simulink model "PMSMdetailTestbench"  (R2022b)
settings: Solver=ode1be  StartTime=0.0  StopTime=400  FixedStep=electricDrive.PmsmControlParams.Ts  RelTol=1e-3  EnableMultiTasking=on
PreLoadFcn:
  | PMSMSystemParamsPopl;
  | load WaterProperties.mat;
  | PMSMthermalParams;
StopFcn:
  | ee_addSimlogTimeStamp(bdroot)
undefined symbols (not defined in the file): electricDrive, p
libraries: fl_lib x71, nesl_utility x25, fl_ps_legacy_lib x23, ee_lib x4, eeTransforms x2, batteryecm_lib x1, autolibshared x1, eePmsmCurrentController x1, eePmsmFwController x1, simulink x1, eePmsmCurrentReferenceGen x1, eeVelocityController x1
(part 1 of 2)
CloseFcn:
  | try,close(h1_ee_pmsm_field_weakening_control),end
  | clear h1_ee_pmsm_field_weakening_control
  | 
  | clear simlogPMSMfocControlLossMaoGen
  | clear logsoutPMSMfocControlLossMaoGen
  | clear air_density alpha beta  Cdc CopperDensity CopperSpHeat CopperThconductivity Cp Cv drag_coefficient dt  gravity h h_conv IronDensity IronSpHeat IronThConductivity Jm k Ld lossMat Lq  max_power max_torque MotorThermal nu p Pmax PmsmControlParams PmsmParams rho  spMat tqMat tout T Tmax  u VehicleParams Vnom
Description:
  | Copyright 2022 - 2023 The MathWorks, Inc.
settings Model: Creator=The MathWorks, Inc.  LastModifiedBy=jjha
settings SolverCC: AlgebraicLoopSolver=TrustRegion  AutoInsertRateTranBlk=on  MaxZcPerStep=1
settings DataIOCC: MaxDataPoints=210000  ReturnWorkspaceOutputs=off  SignalLoggingName=logsoutPMSMfocControlLossMaoGen
settings OptimizationCC: LifeSpan=inf
settings DebuggingCC: UnderspecifiedInitializationDetection=Classic  MergeDetectMultiDrivingBlocksExec=none  UnconnectedInputMsg=warning  UnconnectedOutputMsg=warning  UnconnectedLineMsg=warning  SFUnexpectedBacktrackingDiag=warning  SFNoUnconditionalDefaultTransitionDiag=warning  SFExecutionAtInitializationDiag=none  SFMachineParentedDataDiag=warning  ArithmeticOperatorsInVariantConditions=warning
settings ModelReferenceCC: EnableRefExpFcnMdlSchedulingChecks=on
settings SFSimCC: SimUseLocalCustomCode=off  CustomCodeUndefinedFunction=UseInterfaceOnly
settings RTWCC: RTWUseLocalCustomCode=off  DLArmComputeVersion=19.05
settings CodeAppCC: StateflowObjectComments=on
settings GRTTargetCC: TargetLangStandard=C89/C90 (ANSI)
settings ConfigComp: CovMetricSettings=dw  CovSaveCumulativeToWorkspaceVar=on  CovSaveSingleToWorkspaceVar=on  CovExternalEMLEnable=off
settings SimscapeCC: SimscapeNormalizeSystem=off  SimscapeLogType=all  SimscapeLogSimulationStatistics=on  SimscapeLogName=simlogPMSMdetailTestbench  SimscapeLogDataHistory=700000

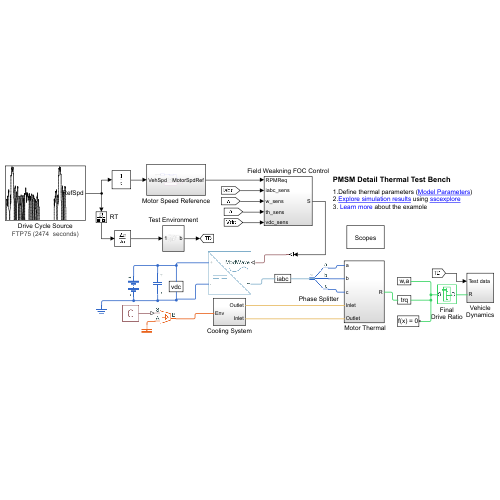
[thumbnail: Simulink's stored preview of the top-level diagram]
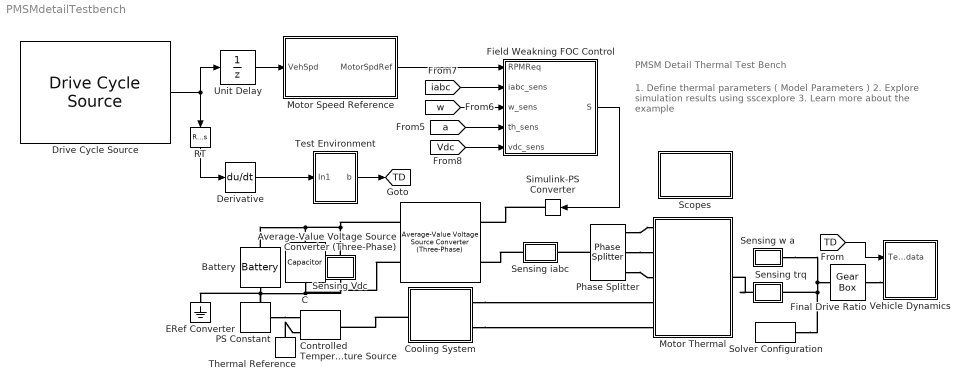
== system PMSMdetailTestbench ==
  note: PMSM Detail Thermal Test Bench
  note: 1. Define thermal parameters ( Model Parameters )
      | 2. Explore simulation results using sscexplore
      | 3. Learn more about the example
  " Motor Thermal" : Subsystem  Tag=PublishSubsystem  VariantControl=Variant1
  Average-Value Voltage Source Converter (Three-Phase) : ee_lib/Semiconductors & Converters/Converters/Average-Value Voltage Source Converter (Three-Phase)  port_option=ee.enum.threePhasePort.composite  frequency_option=ee.enum.converters.frequency.variable  FRated=60 Hz  losses_parameterization=ee.enum.converters.losses.fixed  Pfixed=1 W  ks=0.01  kc1=1.7 V  kc2=0.01 Ohm  Ploss_vect=[100, 800, 1870, 3250, 4900] W  Irms_vect=[10, 100, 200, 300, 400] A  Vdc_nom=300 V  thermal_mass=30000 J/K  temperature_specify=off  temperature_priority=High  temperature=298.15 K  temperature_nominal_specify=off  temperature_nominal_unit=K  temperature_nominal_value=1
      settings: InternalSimscapePortConfiguration="{\"Bottom\":[],\"Left\":[{\"id\":\"ModWave\",\"label\":\"ModWave\",\"type\":\"input\"},{\"id\":\"N\",\"label\":\"~\",\"type\":\"foundation.electrical.three_phase\"}],\"Right\":[{\"id\":\"p\",\"label\":\"+\",\"type\":\"foundation.electrical.electrical\"},{\"id\":\"n\",\"label\":\"-\",\"type\":\"foundation.electrical.electrical\"}],\"Top\":[]}"
  Battery : batteryecm_lib/Battery  Vnom=electricDrive.Vnom V  prm_dir=1  R1_dis=2 Ohm  R1_ch=2 Ohm  R1=0.001 Ohm  prm_AH=simscape.enum.battery.prm_AH.infinite  AH=200 hr*A  V1=290 V  AH1=50 hr*A  prm_R2=1  R2=2000 Ohm  prm_dyn=1  Rp1=0.005 Ohm  tau1=30 s  Rp2=0.005 Ohm  tau2=30 s  Rp3=0.005 Ohm  tau3=30 s  Rp4=0.005 Ohm  tau4=30 s  Rp5=0.005 Ohm  tau5=30 s  prm_fade=1  N_fade=100  AH_fade=45 hr*A  R1_fade=2.02 Ohm  R1_ch_fade=2.02 Ohm  V1_fade=10.35 V  prm_age=1  prm_age_OCV=1  OCV_age=0.9  SOC_age=60  delta_time_age_vec=[0] d  temperature_age_vec=[273] K  OCV_scaling_age=2.2134e6  OCV_offset_age=1.632e6  temp_exp_age=0.515833569 V  t_exp_age=0.75  i_specify=off  i_priority=None  i=0 A  i_nominal_specify=off  i_nominal_unit=A  i_nominal_value=1  v_specify=off  v_priority=None  v=0 V  v_nominal_specify=off  v_nominal_unit=V  v_nominal_value=1  charge_specify=on  charge_priority=High  charge=200 hr*A  charge_nominal_specify=off  charge_nominal_unit=A*hr  charge_nominal_value=1  num_cycles_specify=off  num_cycles_priority=High  num_cycles=0  num_cycles_nominal_specify=off  num_cycles_nominal_unit=1  num_cycles_nominal_value=1  Tmeas=298.15 K  Tmeas_age=298.15 K  Vnom_T2=12 V  R1_T2=2.2 Ohm  R1_T2_dis=2.2 Ohm  R1_T2_ch=2.2 Ohm  V1_T2=11.4 V  R2_T2=2200 Ohm  Rp1_T2=0.005 Ohm  tau1_T2=30 s  Rp2_T2=0.005 Ohm  tau2_T2=30 s  Rp3_T2=0.005 Ohm  tau3_T2=30 s  Rp4_T2=0.005 Ohm  tau4_T2=30 s  Rp5_T2=0.005 Ohm  tau5_T2=30 s  Tmeas2=273.15 K  thermal_mass=30000 J/K  temperature_specify=off  temperature_priority=High  temperature=298.15 K  temperature_nominal_specify=off  temperature_nominal_unit=K  temperature_nominal_value=1
  C : fl_lib/Electrical/Electrical Elements/Capacitor  c=electricDrive.Cdc F  r=1e-6 Ohm  g=0 1/Ohm  i_specify=off  i_priority=None  i=0 A  i_nominal_specify=off  i_nominal_unit=A  i_nominal_value=1  v_specify=off  v_priority=None  v=0 V  v_nominal_specify=off  v_nominal_unit=V  v_nominal_value=1  vc_specify=on  vc_priority=None  vc=electricDrive.Vnom V  vc_nominal_specify=off  vc_nominal_unit=V  vc_nominal_value=1
  Controlled Temperature Source : fl_lib/Thermal/Thermal Sources/Controlled Temperature Source
  Cooling System : Subsystem  Tag=PublishSubsystem
  Derivative : Derivative
  Drive Cycle Source : autolibshared/Drive Cycle Source  cycleVar=FTP75  fileVar=cycleFTP75.mat  tfinal="2474  seconds"  cycleRepeat=off  outAccPort=off  outGearPort=off  gearList=No gear data  t_wot1=5  xdot_woto=0  xdot_wot1=30  t_wot2=20  xdot_wot2=0  t_wotend=30  srcUnit=m/s  outUnit=km/hr  srcAccUnit=m/s/s  outAccUnit=m/s^2  dt=1e-3  aMode=1  faultOption=off  velBnd=2  velBndUnit=mph  inUnit=m/s  timeBnd=1  failOption=off  stopSim=off  maxFaultCnt=10  maxFaultTime=2  maxTotFaultTime=15  traceOption=off  dtTrace=1  traceWindow=10  lastDCname=FTP75  lastOutUnit=mph  lastDT=1e-3  lastTB=1  lastSB=2  forceCalcBound=off
  ERef Converter : fl_lib/Electrical/Electrical Elements/Electrical Reference
  Field Weakning FOC Control : Subsystem
  Final Drive Ratio : fl_lib/Mechanical/Mechanisms/Gear Box  ratio=electricDrive.VehicleParams.Gear_ratio  t_in_specify=off  t_in_priority=High  t_in=0 N*m  t_in_nominal_specify=off  t_in_nominal_unit=N*m  t_in_nominal_value=1  t_out_specify=off  t_out_priority=High  t_out=0 N*m  t_out_nominal_specify=off  t_out_nominal_unit=N*m  t_out_nominal_value=1
  Motor Speed Reference : Subsystem
  PS Constant : fl_lib/Physical Signals/Sources/PS Constant  constant=298.15 K
  Phase Splitter : ee_lib/Connectors & References/Phase Splitter
  RT : RateTransition  OutPortSampleTime=5e-05
  Scopes : Subsystem
      mask Display: disp(get_param(gcb,'Name'))
  Sensing Vdc : Subsystem
      mask Display: disp('vdc')
  Sensing w a : Subsystem
      mask Display: disp('w,a')
  Sensing iabc : Subsystem
      mask Display: disp('iabc')
  Sensing trq : Subsystem
      mask Display: disp('trq')
  Simulink-PS Converter : nesl_utility/Simulink-PS Converter  PhysicalDomain=network_engine_domain  SubClassName=ps_input  LeftPortType=input  RightPortType=output  PseudoPeriodic=off  Frequencies=[]  NoiseDistribution=none  NoiseParameters=[]  Unit=1  AffineConversion=off  FilteringAndDerivatives=provide  SimscapeFilterOrder=1  InputFilterTimeConstant=0.001  UdotUserProvided=0
  Solver Configuration : nesl_utility/Solver Configuration  PhysicalDomain=network_engine_domain  SubClassName=solver  LeftPortType=input  RightPortType=generic  Tones=[]  Harmonics=[]  SimulateNoise=off  Profile=off  UseLocalSampling=off  EnableSwitchedLinearOptims=on  FrequencyDomain=off  UseCCode=off  RelTol=0.001  AbsTol=1e-06  MinStep=1e-09  ToWorkspace=off  RevertToSquareIcSolve=off  NumHomotopyIterations=100  PhasorMode=off  PhasorModeNumHarmonics=1  ConsistencySolver=NEWTON_FTOL  IndexReductionMethod=DerivativeReplacement  DoDC=off  ResidualTolerance=1e-9  ConsistencyTolSource=GLOBAL  ConsistencyAbsTol=0.001  ConsistencyRelTol=0.001  ConsistencyTolFactor=0.001  UseLocalSolver=on  LocalSolverChoice=NE_BACKWARD_EULER_ADVANCER  ResolveIndetEquations=on  FunctionEvalNumThread=1  LocalSolverSampleTime=electricDrive.PmsmControlParams.Ts  DoFixedCost=on  MaxNonlinIter=4  MaxModeIter=2  ComputeImpulses=off  ImpulseIterations=2  LinearAlgebra=auto  LinearAlgebraNumThread=0  EquationFormulation=NE_TIME_EF  DelaysMemoryBudget=1024  AutomaticFiltering=on  FilteringTimeConstant=0.001  PartitionStorageMethod=AS_NEEDED  PartitionMemoryBudget=1024  PartitionMethod=FAST
  Test Environment : Subsystem
  Thermal Reference : fl_lib/Thermal/Thermal Elements/Thermal Reference
  Unit Delay : UnitDelay  SampleTime=-1  HasFrameUpgradeWarning=on
  Vehicle Dynamics : Subsystem
  tag scope: TD=global
  wires:
  Field Weakning FOC Control/1(S) -> Simulink-PS Converter/1
  [Vdc] -> Field Weakning FOC Control/5(vdc_sens)
  [iabc] -> Field Weakning FOC Control/2(iabc_sens)
  [w] -> Field Weakning FOC Control/3(w_sens)
  [a] -> Field Weakning FOC Control/4(th_sens)
  Motor Speed Reference/1(MotorSpdRef) -> Field Weakning FOC Control/1(RPMReq)
  [TD] -> Vehicle Dynamics/1(Test data)
  Drive Cycle Source/1 -> Unit Delay/1, RT/1
  RT/1 -> Derivative/1
  Unit Delay/1 -> Motor Speed Reference/1(VehSpd)
  Derivative/1 -> Test Environment/1(In1)
  Test Environment/1(b) -> [TD]
  connections:
  Sensing Vdc/LConn1 -- Average-Value Voltage Source Converter (Three-Phase)/RConn1 -- Battery/LConn1 -- C/LConn1
  Sensing iabc/LConn1 -- Average-Value Voltage Source Converter (Three-Phase)/LConn2
  Phase Splitter/LConn1 -- Sensing iabc/RConn1
  Sensing trq/LConn1 -- " Motor Thermal"/RConn1
  Battery/RConn1 -- Average-Value Voltage Source Converter (Three-Phase)/RConn2 -- Sensing Vdc/RConn1 -- C/RConn1 -- ERef Converter/LConn1
  Sensing w a/LConn1 -- Solver Configuration/RConn1 -- Sensing trq/RConn1 -- Final Drive Ratio/LConn1
  Phase Splitter/RConn1 -- " Motor Thermal"/LConn1
  Phase Splitter/RConn2 -- " Motor Thermal"/LConn2
  Phase Splitter/RConn3 -- " Motor Thermal"/LConn3
  Final Drive Ratio/RConn1 -- Vehicle Dynamics/LConn1
  Simulink-PS Converter/RConn1 -- Average-Value Voltage Source Converter (Three-Phase)/LConn1
  Cooling System/RConn1 -- " Motor Thermal"/LConn4
  Cooling System/RConn2 -- " Motor Thermal"/LConn5
  Cooling System/LConn1 -- Controlled Temperature Source/LConn1
  PS Constant/RConn1 -- Controlled Temperature Source/RConn1
  Thermal Reference/LConn1 -- Controlled Temperature Source/RConn2

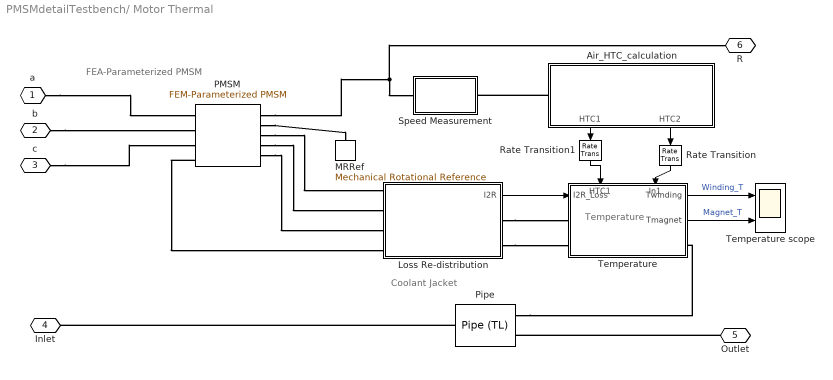
== system PMSMdetailTestbench/ Motor Thermal ==
  note: Temperature
  note: FEA-Parameterized
      | PMSM
  note: Coolant Jacket
  Air_HTC_calculation : Subsystem
      settings: PortSchema="{\"entries\":[{\"content\":{\"sides\":[{\"content\":{\"connectorIds\":[\"LConn1\"]},\"type\":\"ConnectorPlacement.EquallySpacedRectSide\",\"uuid\":\"c3fc49c2-0151-484f-b0d8-f4e4a060bcaf\"},{\"content\":{\"side\":\"RIGHT\"},\"type\":\"ConnectorPlacement.EquallySpacedRectSide\",\"uuid\":\"c73251fe-fcad-4c5f-9d27-fb7ac98c9b31\"},{\"content\":{\"side\":\"TOP\"},\"type\":\"ConnectorPlacement.EquallySpacedRectSide\",\"uuid\":\"06ea8515-c1b4-4445-9ea2-9a6fe3b8d822\"},{\"content\":{\"connectorIds\":[\"Out1\",\"Out2\"],\"side\":\"BOTTOM\"},\"type\":\"ConnectorPlacement.EquallySpacedRectSide\",\"uuid\":\"0d77474d-64a7-49ab-b2b5-eb3962b26dfa\"}]},\"type\":\"ConnectorPlacement.EquallySpacedConnector\",\"uuid\":\"651eda7a-2416-4496-9b8b-1b2d725cf6dd\"}],\"packageUris\":[\"http://schema.mathworks.com/mf0/Connector/R2020b\"],\"version\":\"1.0\"}"
  Loss Re-distribution : Subsystem
  MRRef : fl_lib/Mechanical/Rotational Elements/Mechanical Rotational Reference
  PMSM : ee_lib/Electromechanical/Permanent Magnet/FEM-Parameterized PMSM  parameterization=1  winding_type=ee.enum.statorconnection.wye  iVec=[-2, 0, 2] A  xVec=[0, 20, 40, 60] deg  dfluxdiMatrix=0.0002 * ones(3, 4) Wb/A  dfluxdxMatrix=[0, -.16, .16, 0; 0, -.16, .16, 0; 0, -.16, .16, 0] Wb/rad  calculate_torque_matrix=1  TorqueMatrix=zeros(3, 3, 3, 4) N*m  idVec1=[-200, 0, 200] A  iqVec1=[-200, 0, 200] A  LdMatrix=0.0002 * ones(3, 3) H  LqMatrix=0.0002 * ones(3, 3) H  PmMatrix=0.1 * ones(3, 3) Wb  N=6  interp_method=simscape.enum.interpolation.linear  Rs=electricDrive.PmsmParams.StatorResistance Ohm  Ms=0.00002 H  L0=0.00016 H  loss_param=ee.enum.fem_motor.ironLossesExtended.tabulated  losses_oc=[0, 0, 0] W  losses_sc=[0, 0, 0] W  f_losses=100 % dummy value, not required Hz  Isc_losses=95 A  Inertia=electricDrive.PmsmParams.RotorInertia kg*m^2  lam=0 N*m/(rad/s)  i_d_specify=off  i_d_priority=High  i_d=0 A  i_d_nominal_specify=off  i_d_nominal_unit=A  i_d_nominal_value=1  i_q_specify=off  i_q_priority=High  i_q=0 A  i_q_nominal_specify=off  i_q_nominal_unit=A  i_q_nominal_value=1  torque_specify=off  torque_priority=None  torque=0 N*m  torque_nominal_specify=off  torque_nominal_unit=N*m  torque_nominal_value=1  angular_velocity_specify=off  angular_velocity_priority=High  angular_velocity=PmsmParams.InitialRotorSpeed_rpm rpm  angular_velocity_nominal_specify=off  angular_velocity_nominal_unit=rpm  angular_velocity_nominal_value=1  angular_position_specify=on  angular_position_priority=High  angular_position=electricDrive.PmsmParams.InitialRotorAngle_rad rad  angular_position_nominal_specify=off  angular_position_nominal_unit=deg  angular_position_nominal_value=1  Tmeas=283.15 K  alpha=0.00386 1/K  alpha_flux=-0.001 1/K  stator_thermal_mass=electricDrive.MotorThermal.PhaseWindingThMass J/K  stator_initial_temperatures=[298.15, 298.15, 298.15] K  rotor_thermal_mass=electricDrive.MotorThermal.RotorThMass J/K  rotor_initial_temperature=298.15 K  Rm_percent_rotor=90  Rd_percent_rotor=30  idVec=[-200, 0, 200] A  iqVec=[-200, 0, 200] A  dfluxAdiaMatrix3D=zeros(3, 3, 4) Wb/A  dfluxAdibMatrix3D=zeros(3, 3, 4) Wb/A  dfluxAdicMatrix3D=zeros(3, 3, 4) Wb/A  dfluxAdxMatrix3D=zeros(3, 3, 4) Wb/rad  TorqueMatrix3D=zeros(3, 3, 4) N*m  iaVec=[-200, 0, 200] A  ibVec=[-200, 0, 200] A  icVec=[-200, 0, 200] A  dfluxAdiaMatrix=zeros(3, 3, 3, 4) Wb/A  dfluxAdibMatrix=zeros(3, 3, 3, 4) Wb/A  dfluxAdicMatrix=zeros(3, 3, 3, 4) Wb/A  dfluxAdxMatrix=zeros(3, 3, 3, 4) Wb/rad  param_dq0=ee.enum.fem_motor.fluxTabulationOption.DQpolar  winding_type_dq0=ee.enum.statorconnection.wye  expose_neutral_port=ee.enum.fem_motor.exposeNeutralPort.no  nPolePairs=electricDrive.PmsmParams.NumPolePairs  parks_type=ee.enum.fem_motor.parksType.QleadsD_AphaseToQaxis  idVec2=[-200, 0, 200] A  iqVec2=[-200, 0, 200] A  magVec2=electricDrive.PmsmParams.CurrMagVec*1.3 A  betaVec2=electricDrive.PmsmParams.CurrAdvAngleVec deg  xVec2=electricDrive.PmsmParams.RotorAngleVec deg  fluxD_dq0=zeros(3, 3, 7) Wb  fluxQ_dq0=zeros(3, 3, 7) Wb  fluxA_dq0=zeros(3, 3, 7) Wb  Torque_dq0=zeros(3, 3, 7) N*m  fluxD_IBX=electricDrive.PmsmParams.FluxDMat Wb  fluxQ_IBX=electricDrive.PmsmParams.FluxQMat Wb  fluxA_IBX=fluxAmat Wb  Torque_IBX=electricDrive.PmsmParams.TorqueMat N*m  rotorLossCoeff_k_h_DQ=zeros(3, 3) W/Hz  rotorLossCoeff_k_J_DQ=zeros(3, 3) W/Hz^2  rotorLossCoeff_k_ex_DQ=zeros(3, 3) W/Hz^(3/2)  rotorLossCoeff_k_h_IB=electricDrive.PmsmParams.RotorKhMat W/Hz  rotorLossCoeff_k_J_IB=electricDrive.PmsmParams.RotorKjMat W/Hz^2  rotorLossCoeff_k_ex_IB=electricDrive.PmsmParams.RotorKexMat W/Hz^(3/2)  statorLossCoeff_k_h_DQ=zeros(3, 3) W/Hz  statorLossCoeff_k_J_DQ=zeros(3, 3) W/Hz^2  statorLossCoeff_k_ex_DQ=zeros(3, 3) W/Hz^(3/2)  statorLossCoeff_k_h_IB=electricDrive.PmsmParams.StatorKhMat W/Hz  statorLossCoeff_k_J_IB=electricDrive.PmsmParams.StatorKjMat W/Hz^2  statorLossCoeff_k_ex_IB=electricDrive.PmsmParams.StatorKexMat W/Hz^(3/2)  wVec=[1000, 2000] rpm  rotorLossTable_DQ=zeros(3, 3, 2) W  rotorLossTable_IB=zeros(3, 5, 2) W  statorLossTable_DQ=zeros(3, 3, 2) W  statorLossTable_IB=zeros(3, 5, 2) W  electrical_torque_before_iron_losses_specify=off  electrical_torque_before_iron_losses_priority=None  electrical_torque_before_iron_losses=0 N*m  electrical_torque_before_iron_losses_nominal_specify=off  electrical_torque_before_iron_losses_nominal_unit=N*m  electrical_torque_before_iron_losses_nominal_value=1  Qrotor_specify=off  Qrotor_priority=None  Qrotor=0 J/s  Qrotor_nominal_specify=off  Qrotor_nominal_unit=J/s  Qrotor_nominal_value=1  Qstator_specify=off  Qstator_priority=None  Qstator=0 J/s  Qstator_nominal_specify=off  Qstator_nominal_unit=J/s  Qstator_nominal_value=1
      settings: InternalSimscapePortConfiguration="{\"Bottom\":[],\"Left\":[{\"id\":\"a\",\"label\":\"a\",\"type\":\"foundation.electrical.electrical\"},{\"id\":\"b\",\"label\":\"b\",\"type\":\"foundation.electrical.electrical\"},{\"id\":\"c\",\"label\":\"c\",\"type\":\"foundation.electrical.electrical\"},{\"id\":\"HR\",\"label\":\"HR\",\"type\":\"foundation.thermal.thermal\"}],\"Right\":[{\"id\":\"R\",\"label\":\"R\",\"type\":\"foundation.mechanical.rotational.rotational\"},{\"id\":\"C\",\"label\":\"C\",\"type\":\"foundation.mechanical.rotational.rotational\"},{\"id\":\"HA\",\"label\":\"HA\",\"type\":\"foundation.thermal.thermal\"},{\"id\":\"HB\",\"label\":\"HB\",\"type\":\"foundation.thermal.thermal\"},{\"id\":\"HC\",\"label\":\"HC\",\"type\":\"foundation.thermal.thermal\"}],\"Top\":[]}"
  Pipe : fl_lib/Thermal Liquid/Elements/Pipe (TL)  length=electricDrive.MotorThermal.ChannelLength mm  area=electricDrive.MotorThermal.ChannelSection mm^2  Dh=electricDrive.MotorThermal.ChannelHydraulicdia mm  length_add=500 mm  roughness=1.5e-5 m  Re_lam=2e+3  Re_tur=4e+3  shape_factor=64  Nu_lam=3.66  dynamic_compressibility=1  inertia=0  p0=1 atm  T0=298.15 K  mdot0=0.1 kg/s
  Rate Transition : RateTransition
  Rate Transition1 : RateTransition
  Speed Measurement : Subsystem
  Temperature : Subsystem
      settings: PortSchema="{\"entries\":[{\"content\":{\"sides\":[{\"content\":{\"connectorIds\":[\"In1\",\"LConn1\",\"LConn2\"]},\"type\":\"ConnectorPlacement.EquallySpacedRectSide\",\"uuid\":\"fee72484-960d-4cd4-9296-e38678962aa1\"},{\"content\":{\"connectorIds\":[\"Out1\",\"Out2\",\"RConn1\"],\"side\":\"RIGHT\"},\"type\":\"ConnectorPlacement.EquallySpacedRectSide\",\"uuid\":\"5fc115b4-63fd-47d3-871d-1c82ac52ac43\"},{\"content\":{\"connectorIds\":[\"In2\",\"In3\"],\"side\":\"TOP\"},\"type\":\"ConnectorPlacement.EquallySpacedRectSide\",\"uuid\":\"406f719a-f995-4122-9f35-24e8332a2e84\"},{\"content\":{\"side\":\"BOTTOM\"},\"type\":\"ConnectorPlacement.EquallySpacedRectSide\",\"uuid\":\"14dc85e6-8157-4b38-8651-862ce77721cd\"}]},\"type\":\"ConnectorPlacement.EquallySpacedConnector\",\"uuid\":\"1dcc2b5d-90fd-40de-873d-99118eb86bdd\"}],\"packageUris\":[\"http://schema.mathworks.com/mf0/Connector/R2020b\"],\"version\":\"1.0\"}"
  Temperature scope : Scope  NumInputPorts=2
  a : PMIOPort  Side=Left
  b : PMIOPort  Port=2  Side=Left
  c : PMIOPort  Port=3  Side=Left
  Inlet : PMIOPort  Port=4  Side=Left
  Outlet : PMIOPort  Port=5  Side=Left
  R : PMIOPort  Port=6  Side=Right
  wires:
  Temperature/1(Twinding) -> Temperature scope/1  "Winding_T"
  Temperature/2(Tmagnet) -> Temperature scope/2  "Magnet_T"
  Loss Re-distribution/1(I2R) -> Temperature/1(I2R_Loss)
  Rate Transition/1 -> Temperature/3(In1)
  Air_HTC_calculation/2(HTC2) -> Rate Transition/1
  Air_HTC_calculation/1(HTC1) -> Rate Transition1/1
  Rate Transition1/1 -> Temperature/2(HTC1)
  connections:
  b/RConn1 -- PMSM/LConn2
  Pipe/RConn1 -- Inlet/RConn1
  PMSM/RConn2 -- MRRef/LConn1
  PMSM/RConn1 -- R/RConn1 -- Speed Measurement/LConn1
  Outlet/RConn1 -- Pipe/LConn1
  a/RConn1 -- PMSM/LConn1
  Air_HTC_calculation/LConn1 -- Speed Measurement/RConn1
  Pipe/LConn2 -- Temperature/RConn1
  Loss Re-distribution/RConn1 -- Temperature/LConn1
  Loss Re-distribution/RConn2 -- Temperature/LConn2
  c/RConn1 -- PMSM/LConn3
  PMSM/LConn4 -- Loss Re-distribution/LConn4
  PMSM/RConn3 -- Loss Re-distribution/LConn1
  PMSM/RConn4 -- Loss Re-distribution/LConn2
  PMSM/RConn5 -- Loss Re-distribution/LConn3

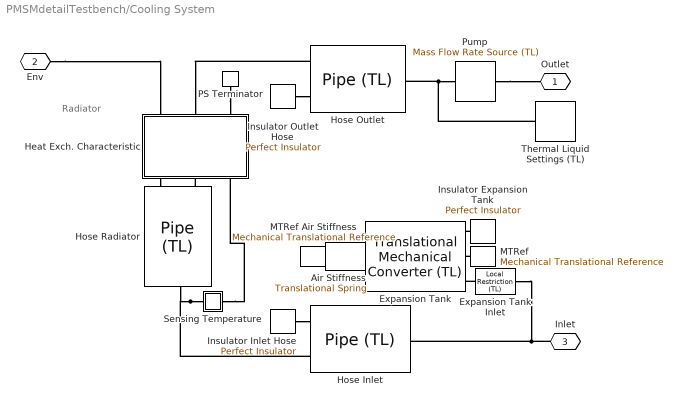
== system PMSMdetailTestbench/Cooling System ==
  note: Radiator
  Air Stiffness : fl_lib/Mechanical/Translational Elements/Translational Spring  spr_rate=1e3 N/m  v_specify=off  v_priority=High  v=0 m/s  v_nominal_specify=off  v_nominal_unit=m/s  v_nominal_value=1  f_specify=on  f_priority=Low  f=0 N  f_nominal_specify=off  f_nominal_unit=N  f_nominal_value=1  x_specify=off  x_priority=High  x=0 m  x_nominal_specify=off  x_nominal_unit=m  x_nominal_value=1
  Expansion Tank : fl_lib/Thermal Liquid/Elements/Translational Mechanical Converter (TL)  mech_orientation=1  displacement_spec=foundation.enum.DisplacementSpec.Calculate  x0=200 mm  interface_area=pi*50^2 mm^2  dead_volume=0.01 m^3  environment_spec=1  environment_pressure=0.101325 MPa  dynamic_compressibility=0  p0=1 atm  T0=298.15 K
      settings: InternalSimscapePortConfiguration="{\"Bottom\":[],\"Left\":[{\"id\":\"A\",\"label\":\"A\",\"type\":\"foundation.thermal_liquid.thermal_liquid\"},{\"id\":\"C\",\"label\":\"C\",\"type\":\"foundation.mechanical.translational.translational\"},{\"id\":\"H\",\"label\":\"H\",\"type\":\"foundation.thermal.thermal\"}],\"Right\":[{\"id\":\"R\",\"label\":\"R\",\"type\":\"foundation.mechanical.translational.translational\"}],\"Top\":[]}"
  Expansion Tank Inlet : fl_lib/Thermal Liquid/Elements/Local Restriction (TL)  restriction_type=foundation.enum.restriction_type.fixed  restriction_area=pi*10^2 mm^2  min_area=1e-10 m^2  max_area=0.005 m^2  area=pi*11^2 mm^2  Cd=0.7  pressure_recovery=0  Re_c=12
  Heat Exch. Characteristic : Subsystem
  Hose Radiator : fl_lib/Thermal Liquid/Elements/Pipe (TL)  length=1000 mm  area=pi*100^2 mm^2  Dh=50 mm  length_add=500 mm  roughness=1.5e-5 m  Re_lam=2e+3  Re_tur=4e+3  shape_factor=64  Nu_lam=3.66  dynamic_compressibility=1  inertia=0  p0=1 atm  T0=298.15 K  mdot0=0.1 kg/s
  Hose Inlet : fl_lib/Thermal Liquid/Elements/Pipe (TL)  length=50 mm  area=pi*100^2 mm^2  Dh=200 mm  length_add=500 mm  roughness=1.5e-5 m  Re_lam=2e+3  Re_tur=4e+3  shape_factor=64  Nu_lam=3.66  dynamic_compressibility=1  inertia=0  p0=1 atm  T0=298.15 K  mdot0=0.1 kg/s
  Hose Outlet : fl_lib/Thermal Liquid/Elements/Pipe (TL)  length=50 mm  area=pi*100^2 mm^2  Dh=200 mm  length_add=500 mm  roughness=1.5e-5 m  Re_lam=2e+3  Re_tur=4e+3  shape_factor=64  Nu_lam=3.66  dynamic_compressibility=1  inertia=0  p0=1 atm  T0=298.15 K  mdot0=0.1 kg/s
  Insulator Expansion Tank : fl_lib/Thermal/Thermal Elements/Perfect Insulator  T_specify=off  T_priority=High  T=0 K  T_nominal_specify=off  T_nominal_unit=K  T_nominal_value=1
  Insulator Inlet Hose : fl_lib/Thermal/Thermal Elements/Perfect Insulator  T_specify=off  T_priority=High  T=0 K  T_nominal_specify=off  T_nominal_unit=K  T_nominal_value=1
  Insulator Outlet Hose : fl_lib/Thermal/Thermal Elements/Perfect Insulator  T_specify=off  T_priority=High  T=0 K  T_nominal_specify=off  T_nominal_unit=K  T_nominal_value=1
  MTRef : fl_lib/Mechanical/Translational Elements/Mechanical Translational Reference
  MTRef Air Stiffness : fl_lib/Mechanical/Translational Elements/Mechanical Translational Reference
  PS Terminator : fl_lib/Physical Signals/Sinks/PS Terminator
  Pump : fl_lib/Thermal Liquid/Sources/Mass Flow Rate Source (TL)  commanded_mass_flow=0.13 kg/s  area=pi*100^2 mm^2
      settings: InternalSimscapePortConfiguration="{\"Bottom\":[],\"Left\":[{\"id\":\"A\",\"label\":\"A\",\"type\":\"foundation.thermal_liquid.thermal_liquid\"}],\"Right\":[{\"id\":\"B\",\"label\":\"B\",\"type\":\"foundation.thermal_liquid.thermal_liquid\"}],\"Top\":[]}"
  Sensing Temperature : Subsystem
      mask Display: disp('T')
  Thermal Liquid Settings (TL) : fl_lib/Thermal Liquid/Utilities/Thermal Liquid Settings (TL)  table_dimensions=foundation.enum.table_dimensions_TL.two_dimensional  T_TLU=T K  p_TLU=p Pa  p_atm=1 atm  pT_region_flag=foundation.enum.pT_region_TL.min_max  T_min=273.16 K  T_max=373.16 K  p_min=p(1) Pa  p_max=p(end) Pa  T_min_1D=273.16 K  T_max_1D=373.16 K  p_min_1D=0.01 MPa  p_max_1D=50 MPa  pT_validity_TLU=ones(11, 12)  rho_parameterization_2D=foundation.enum.rho_parameterization_2D.rho_beta_alpha  rho_parameterization_1D=foundation.enum.rho_parameterization_1D.rho_vector  rho_TLU=rho kg/m^3  beta_TLU=beta Pa  alpha_TLU=alpha 1/K  rho_TLU_2=[999.7973, 999.8431, 1002.3216, 1004.8218, 1007.293, 1009.7358, 1012.1506, 1014.5379, 1016.8979, 1019.2311, 1021.538, 1023.8188; 999.6579, 999.7009, 1002.0303, 1004.382, 1006.7084, 1009.0101, 1011.2874, 1013.5407, 1015.7703, 1017.9766, 1020.1599, 1022.3206; 998.1632, 998.2045, 1000.4375, 1002.6924, 1004.9239, 1007.1324, 1009.3183, 1011.4819, 1013.6236, 1015.7438, 1017.8428, 1019.921; 995.6057, 995.6458, 997.81864, 1000.0128, 1002.1841, 1004.3332, 1006.4603, 1008.566, 1010.6505, 1012.7144, 1014.758, 1016.7815; 992.1724, 992.2119, 994.35133, 996.5113, 998.6484, 1000.7633, 1002.8563, 1004.928, 1006.9788, 1009.009, 1011.0192, 1013.0097; 988.02, 988.0299, 990.15684, 992.3035, 994.4268, 996.5273, 998.6056, 1000.6622, 1002.6976, 1004.7123, 1006.7067, 1008.6813; 983.18, 983.1901, 985.3217, 987.4721, 989.5983, 991.7008, 993.7803, 995.8374, 997.8726, 999.8864, 1001.8795, 1003.8522; 977.75, 977.7583, 979.9094, 982.0783, 984.2216, 986.34, 988.4343, 990.505, 992.5529, 994.5786, 996.5825, 998.5654; 971.77, 971.7836, 973.96734, 976.1678, 978.3409, 980.4876, 982.6087, 984.7049, 986.7768, 988.8254, 990.8511, 992.8545; 965.26, 965.3023, 967.53107, 969.7753, 971.9901, 974.1764, 976.3354, 978.4676, 980.5741, 982.6556, 984.7129, 986.7465; 958.62, 958.6315, 960.627, 962.9267, 965.1944, 967.4314, 969.6387, 971.8173, 973.9681, 976.0921, 978.19, 980.2628] kg/m^3  rho_ref_3=998.21 kg/m^3  T_ref_3=293.16 K  p_ref_3=0.101325 MPa  beta_const_3=2.1791 GPa  alpha_const_3=2.0691e-4 1/K  rho_TLU_4=[999.84; 999.7; 998.2; 995.65; 992.21; 988.03; 983.19; 977.76; 971.78; 965.3; 958.8] kg/m^3  beta_const_4=2.1791 GPa  p_ref_4=0.101325 MPa  rho_ref_5=998.21 kg/m^3  T_ref_5=293.16 K  p_ref_5=0.101325 MPa  beta_const_5=2.1791 GPa  alpha_const_5=2.0691e-4 1/K  u_parameterization_2D=foundation.enum.u_parameterization_2D.u_cp  u_parameterization_1D=foundation.enum.u_parameterization_1D.u  u_TLU=u J/g  cp_TLU=Cp J/K/g  u_TLU_2=[.0002, .0018, .086, .1588, .219, .267, .3034, .3288, .3436, .3483, .3435, .3294; 42.062, 42.06, 41.935, 41.804, 41.668, 41.527, 41.382, 41.233, 41.081, 40.924, 40.763, 40.599; 83.953, 83.948, 83.651, 83.349, 83.049, 82.749, 82.451, 82.153, 81.856, 81.56, 81.265, 80.971; 125.77, 125.76, 125.31, 124.86, 124.41, 123.97, 123.53, 123.1, 122.68, 122.25, 121.84, 121.42; 167.57, 167.56, 166.96, 166.37, 165.79, 165.21, 164.65, 164.09, 163.54, 163, 162.46, 161.94; 209.36, 209.36, 208.63, 207.9, 207.19, 206.48, 205.79, 205.11, 204.45, 203.79, 203.14, 202.5; 251.19, 251.19, 250.33, 249.47, 248.62, 247.79, 246.98, 246.18, 245.39, 244.62, 243.86, 243.12; 293.06, 293.06, 292.07, 291.07, 290.1, 289.14, 288.2, 287.28, 286.38, 285.49, 284.62, 283.77; 334.99, 334.99, 333.86, 332.73, 331.63, 330.54, 329.48, 328.44, 327.41, 326.41, 325.43, 324.46; 377, 377, 375.73, 374.46, 373.22, 372, 370.81, 369.64, 368.5, 367.38, 366.27, 365.19; 419.01, 419.01, 417.69, 416.27, 414.89, 413.54, 412.21, 410.91, 409.64, 408.4, 407.17, 405.98] kJ/kg  cp_TLU_3=[4.2199, 4.2194, 4.1957, 4.1726, 4.1508, 4.13, 4.1103, 4.0916, 4.0738, 4.0569, 4.0408, 4.0254; 4.1955, 4.1951, 4.1769, 4.1592, 4.1422, 4.1259, 4.1103, 4.0954, 4.0812, 4.0676, 4.0545, 4.0421; 4.1843, 4.184, 4.169, 4.1543, 4.1401, 4.1264, 4.1133, 4.1007, 4.0885, 4.0768, 4.0656, 4.0548; 4.1801, 4.1798, 4.1667, 4.1538, 4.1413, 4.1293, 4.1177, 4.1064, 4.0956, 4.0851, 4.075, 4.0653; 4.1796, 4.1794, 4.1675, 4.1558, 4.1444, 4.1334, 4.1227, 4.1123, 4.1023, 4.0926, 4.0832, 4.0741; 4.1813, 4.1813, 4.1702, 4.1592, 4.1484, 4.138, 4.1279, 4.1181, 4.1086, 4.0993, 4.0903, 4.0816; 4.185, 4.185, 4.1742, 4.1636, 4.1532, 4.1432, 4.1334, 4.1239, 4.1146, 4.1056, 4.0969, 4.0884; 4.1901, 4.1901, 4.1795, 4.169, 4.1588, 4.1489, 4.1393, 4.1299, 4.1207, 4.1118, 4.1032, 4.0947; 4.1968, 4.1968, 4.1862, 4.1757, 4.1655, 4.1555, 4.1458, 4.1364, 4.1273, 4.1183, 4.1096, 4.1012; 4.2052, 4.2052, 4.1944, 4.1837, 4.1733, 4.1632, 4.1534, 4.1438, 4.1345, 4.1255, 4.1166, 4.108; 4.2136, 4.2136, 4.2045, 4.1935, 4.1828, 4.1724, 4.1623, 4.1524, 4.1429, 4.1335, 4.1245, 4.1157] kJ/kg/K  u_TLU_4=[.0018; 42.06; 83.948; 125.76; 167.56; 209.36; 251.19; 293.06; 334.99; 377; 418.01] kJ/kg  cp_TLU_5=[4.2199; 4.1955; 4.1843; 4.1801; 4.1796; 4.1813; 4.185; 4.1901; 4.1968; 4.2052; 4.2136] kJ/kg/K  nu_TLU=nu cm^2/s  nu_TLU_2=[1.7917; 1.3061; 1.0032; .8006; .6577; .553; .4739; .4127; .3643; .3254; .2866] mm^2/s  k_TLU=k mW/m/K  k_TLU_2=[561.04; 580.02; 598.44; 615.48; 630.6; 643.61; 654.39; 663.13; 670.02; 675.27; 680.52] mW/m/K
  Outlet : PMIOPort  Side=Right
  Env : PMIOPort  Port=2  Side=Left
  Inlet : PMIOPort  Port=3  Side=Right
  connections:
  Insulator Outlet Hose/LConn1 -- Hose Outlet/LConn2
  Insulator Inlet Hose/LConn1 -- Hose Inlet/LConn2
  Env/RConn1 -- Heat Exch. Characteristic/RConn1
  Thermal Liquid Settings (TL)/RConn1 -- Hose Outlet/RConn1 -- Pump/LConn1
  Hose Outlet/LConn1 -- Heat Exch. Characteristic/RConn2
  Pump/RConn1 -- Outlet/RConn1
  Inlet/RConn1 -- Expansion Tank Inlet/LConn1 -- Hose Inlet/RConn1
  Sensing Temperature/LConn1 -- Hose Radiator/RConn1 -- Hose Inlet/LConn1
  Hose Radiator/LConn1 -- Heat Exch. Characteristic/LConn2
  Heat Exch. Characteristic/LConn1 -- Hose Radiator/LConn2
  Sensing Temperature/RConn1 -- Heat Exch. Characteristic/LConn3
  PS Terminator/LConn1 -- Heat Exch. Characteristic/RConn3
  Insulator Expansion Tank/LConn1 -- Expansion Tank/LConn3
  Air Stiffness/RConn1 -- MTRef Air Stiffness/LConn1
  Air Stiffness/LConn1 -- Expansion Tank/RConn1
  Expansion Tank Inlet/RConn1 -- Expansion Tank/LConn1
  MTRef/LConn1 -- Expansion Tank/LConn2

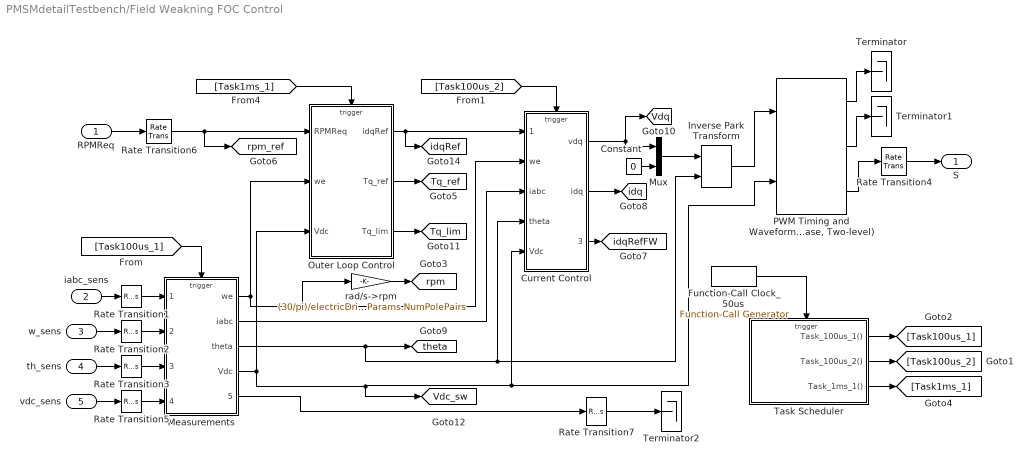
== system PMSMdetailTestbench/Field Weakning FOC Control ==
  RPMReq : Inport
  iabc_sens : Inport  Port=2
  w_sens : Inport  Port=3
  th_sens : Inport  Port=4
  vdc_sens : Inport  Port=5
  Constant : Constant  Value=0  SampleTime=-1
  Current Control : Subsystem
  Function-Call Clock_50us : simulink/Ports & Subsystems/Function-Call Generator  sample_time=1e-4  numberOfIterations=1  DisallowWideOutput=off
  Inverse Park Transform : eeTransforms/Inverse Park Transform  AxisAlignment=Q-axis  PowerInvariant=off
  Measurements : Subsystem
  Mux : Mux  Inputs=2
  Outer Loop Control : Subsystem
  "PWM Timing and Waveform Generator (Three-phase, Two-level)" : eePwmGeneratorTwoLevel/PWM Timing and Waveform Generator (Three-phase, Two-level)  PWMMode=Continuous PWM (CPWM)  CPWMMode=SVM: space vector modulation  DPWMMode=60 DPWM (-30 degree shift): -30 degree shift from 60 DPWM  fsw=1e4
      settings: SamplingMode=Natural
  Rate Transition{1..7} (7 alike) : RateTransition
  Task Scheduler : Stateflow chart  TreatAsAtomicUnit=on
  Terminator : Terminator
  Terminator1 : Terminator
  Terminator2 : Terminator
  rad/s->rpm : Gain  Gain=(30/pi)/electricDrive.PmsmParams.NumPolePairs
  S : Outport  VectorParamsAs1DForOutWhenUnconnected=off
  tag scope: Tq_lim=global, Tq_ref=global, Vdc_sw=global, Vdq=global, idq=global, idqRef=global, idqRefFW=global, rpm=global, rpm_ref=global, theta=global
  wires:
  [Task100us_1] -> Measurements/Trigger
  [Task100us_2] -> Current Control/Trigger
  Current Control/1(vdq) -> Mux/1, [Vdq]
  Measurements/2(iabc) -> Current Control/3(iabc)
  Measurements/3(theta) -> Inverse Park Transform/2, Current Control/4(theta), [theta]
  Inverse Park Transform/1 -> "PWM Timing and Waveform Generator (Three-phase, Two-level)"/1
  iabc_sens/1 -> Rate Transition1/1
  w_sens/1 -> Rate Transition2/1
  th_sens/1 -> Rate Transition3/1
  vdc_sens/1 -> Rate Transition5/1
  RPMReq/1 -> Rate Transition6/1
  Rate Transition1/1 -> Measurements/1(iabc_sens)
  Rate Transition2/1 -> Measurements/2(w_sens)
  Rate Transition3/1 -> Measurements/3(th_sens)
  Rate Transition5/1 -> Measurements/4(Vdc_sens)
  Rate Transition6/1 -> [rpm_ref], Outer Loop Control/1(RPMReq)
  Measurements/4(Vdc) -> [Vdc_sw], "PWM Timing and Waveform Generator (Three-phase, Two-level)"/2, Current Control/5(Vdc), Outer Loop Control/3(Vdc)
  Function-Call Clock_50us/1 -> Task Scheduler/Trigger
  Task Scheduler/3(Task_1ms_1()) -> [Task1ms_1]
  Task Scheduler/2(Task_100us_2()) -> [Task100us_2]
  Task Scheduler/1(Task_100us_1()) -> [Task100us_1]
  Outer Loop Control/2(Tq_ref) -> [Tq_ref]
  Measurements/1(we) -> Current Control/2(we), rad/s->rpm/1, Outer Loop Control/2(we)
  rad/s->rpm/1 -> [rpm]
  Current Control/2(idq) -> [idq]
  Outer Loop Control/3(Tq_lim) -> [Tq_lim]
  Rate Transition4/1 -> S/1
  Measurements/5(PwmEnable) -> Rate Transition7/1
  [Task1ms_1] -> Outer Loop Control/Trigger
  Mux/1 -> Inverse Park Transform/1
  Constant/1 -> Mux/2
  Outer Loop Control/1(idqRef) -> Current Control/1(idq_ref), [idqRef]
  Current Control/3(idqRefFW) -> [idqRefFW]
  "PWM Timing and Waveform Generator (Three-phase, Two-level)"/1 -> Terminator/1
  "PWM Timing and Waveform Generator (Three-phase, Two-level)"/3 -> Rate Transition4/1
  "PWM Timing and Waveform Generator (Three-phase, Two-level)"/2 -> Terminator1/1
  Rate Transition7/1 -> Terminator2/1

== system PMSMdetailTestbench/Motor Speed Reference ==
  VehSpd : Inport  Unit=km/hr
  Constant1 : Constant  Value=electricDrive.VehicleParams.wheel_radius
  Divide : Product  Inputs=*/
  Gain : Gain  Gain=2*pi
  Gear_ratio : Constant  Value=electricDrive.VehicleParams.Gear_ratio
  Product : Product
  Signal Specification : SignalSpecification  Unit=m/min
  Unit Conversion : UnitConversion
  MotorSpdRef : Outport  Unit=rpm  VectorParamsAs1DForOutWhenUnconnected=off
  wires:
  VehSpd/1 -> Unit Conversion/1
  Unit Conversion/1 -> Signal Specification/1
  Signal Specification/1 -> Divide/1
  Gain/1 -> Divide/2  "2*pi*R (m)"
  Divide/1 -> Product/1  "tireRpmRef"
  Gear_ratio/1 -> Product/2
  Product/1 -> MotorSpdRef/1  "motorRpmRef"
  Constant1/1 -> Gain/1  "m"

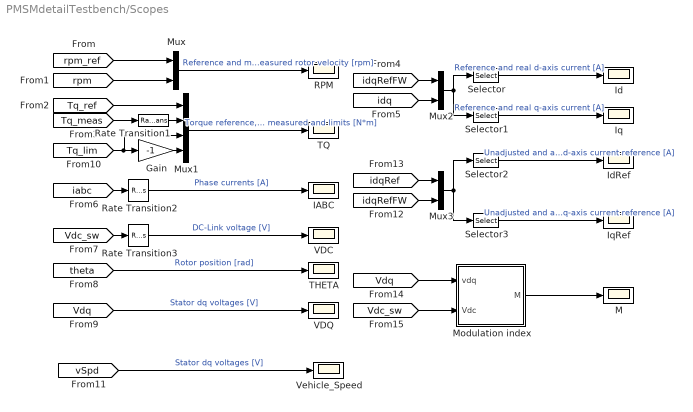
== system PMSMdetailTestbench/Scopes ==
  Gain : Gain  Gain=-1
  IABC : Scope
  Id : Scope
  IdRef : Scope
  Iq : Scope
  IqRef : Scope
  M : Scope
  Modulation index : Subsystem
  Mux : Mux  Inputs=2
  Mux1 : Mux
  Mux2 : Mux  Inputs=2
  Mux3 : Mux  Inputs=2
  RPM : Scope
  Rate Transition1 : RateTransition
  Rate Transition2 : RateTransition  OutPortSampleTime=1e-4
  Rate Transition3 : RateTransition  OutPortSampleTime=1e-4
  Selector : Selector  InputPortWidth=4  IndexOptions=Index vector (dialog)  Indices=[1 3]  OutputSizes=1
  Selector1 : Selector  InputPortWidth=4  IndexOptions=Index vector (dialog)  Indices=[2 4]  OutputSizes=1
  Selector2 : Selector  InputPortWidth=4  IndexOptions=Index vector (dialog)  Indices=[1 3]  OutputSizes=1
  Selector3 : Selector  InputPortWidth=4  IndexOptions=Index vector (dialog)  Indices=[2 4]  OutputSizes=1
  THETA : Scope
  TQ : Scope
  VDC : Scope
  VDQ : Scope
  Vehicle_Speed : Scope
  wires:
  [rpm] -> Mux/2
  Selector1/1 -> Iq/1  "Reference and real q-axis current [A]"
  Mux2/1 -> Selector1/1, Selector/1
  Gain/1 -> Mux1/4
  Rate Transition3/1 -> VDC/1  "DC-Link voltage [V]"
  [Vdc_sw] -> Rate Transition3/1
  [idqRefFW] -> Mux2/1
  [Tq_ref] -> Mux1/1
  Rate Transition2/1 -> IABC/1  "Phase currents [A]"
  [idq] -> Mux2/2
  [rpm_ref] -> Mux/1
  [iabc] -> Rate Transition2/1
  [Tq_meas] -> Rate Transition1/1
  [Vdq] -> VDQ/1  "Stator dq voltages [V]"
  Selector/1 -> Id/1  "Reference and real d-axis current [A]"
  [Tq_lim] -> Mux1/3, Gain/1
  Mux1/1 -> TQ/1  "Torque reference, measured and limits [N*m]"
  [theta] -> THETA/1  "Rotor position [rad]"
  Rate Transition1/1 -> Mux1/2
  Mux/1 -> RPM/1  "Reference and measured rotor velocity [rpm]"
  Selector2/1 -> IdRef/1  "Unadjusted and adjusted d-axis current reference [A]"
  Mux3/1 -> Selector2/1, Selector3/1
  Selector3/1 -> IqRef/1  "Unadjusted and adjusted q-axis current reference [A]"
  [idqRefFW] -> Mux3/2
  [idqRef] -> Mux3/1
  [Vdq] -> Modulation index/1(vdq)
  [Vdc_sw] -> Modulation index/2(Vdc)
  Modulation index/1(M) -> M/1
  [vSpd] -> Vehicle_Speed/1  "Stator dq voltages [V]"

== system PMSMdetailTestbench/Sensing Vdc ==
  PS-Simulink Converter4 : nesl_utility/PS-Simulink Converter  PhysicalDomain=network_engine_domain  SubClassName=ps_output  LeftPortType=input  RightPortType=output  PseudoPeriodic=off  Frequencies=[]  VectorFormat=1-D array  Unit=V  AffineConversion=off
  Voltage Sensor : fl_lib/Electrical/Electrical Sensors/Voltage Sensor
  + : PMIOPort  Side=Left
  - : PMIOPort  Port=2  Side=Right
  tag scope: Vdc=global
  wires:
  PS-Simulink Converter4/1 -> [Vdc]
  connections:
  Voltage Sensor/LConn1 -- +/RConn1
  Voltage Sensor/RConn2 -- -/RConn1
  PS-Simulink Converter4/LConn1 -- Voltage Sensor/RConn1

== system PMSMdetailTestbench/Sensing w a ==
  MRRef : fl_lib/Mechanical/Rotational Elements/Mechanical Rotational Reference
  Motion Sensor : fl_lib/Mechanical/Mechanical Sensors/Ideal Rotational Motion Sensor  reference=foundation.enum.MeasurementReference.difference  acceleration_port=false  velocity_port=true  position_port=true  wrap_angle=simscape.enum.onoff.off  offset=0 deg
  PS-Simulink Converter1 : nesl_utility/PS-Simulink Converter  PhysicalDomain=network_engine_domain  SubClassName=ps_output  LeftPortType=input  RightPortType=output  PseudoPeriodic=off  Frequencies=[]  VectorFormat=1-D array  Unit=rad/s  AffineConversion=off
  PS-Simulink Converter2 : nesl_utility/PS-Simulink Converter  PhysicalDomain=network_engine_domain  SubClassName=ps_output  LeftPortType=input  RightPortType=output  PseudoPeriodic=off  Frequencies=[]  VectorFormat=1-D array  Unit=rad  AffineConversion=off
  R : PMIOPort  Side=Left
  tag scope: a=global, w=global
  wires:
  PS-Simulink Converter1/1 -> [w]
  PS-Simulink Converter2/1 -> [a]
  connections:
  R/RConn1 -- Motion Sensor/LConn1
  Motion Sensor/RConn2 -- PS-Simulink Converter1/LConn1
  MRRef/LConn1 -- Motion Sensor/RConn1
  Motion Sensor/RConn3 -- PS-Simulink Converter2/LConn1

== system PMSMdetailTestbench/Sensing iabc ==
  Current Sensor : ee_lib/Sensors & Transducers/Current Sensor (Three-Phase)
  PS-Simulink Converter : nesl_utility/PS-Simulink Converter  PhysicalDomain=network_engine_domain  SubClassName=ps_output  LeftPortType=input  RightPortType=output  PseudoPeriodic=off  Frequencies=[]  VectorFormat=1-D array  Unit=A  AffineConversion=off
  1 : PMIOPort  Side=Left
  2 : PMIOPort  Port=2  Side=Right
  tag scope: iabc=global
  wires:
  PS-Simulink Converter/1 -> [iabc]
  connections:
  1/RConn1 -- Current Sensor/LConn1
  2/RConn1 -- Current Sensor/RConn2
  Current Sensor/RConn1 -- PS-Simulink Converter/LConn1

== system PMSMdetailTestbench/Sensing trq ==
  PS-Simulink Converter3 : nesl_utility/PS-Simulink Converter  PhysicalDomain=network_engine_domain  SubClassName=ps_output  LeftPortType=input  RightPortType=output  PseudoPeriodic=off  Frequencies=[]  VectorFormat=1-D array  Unit=N*m  AffineConversion=off
  Torque Sensor : fl_lib/Mechanical/Mechanical Sensors/Ideal Torque Sensor
  R : PMIOPort  Side=Left
  C : PMIOPort  Port=2  Side=Right
  tag scope: Tq_meas=global
  wires:
  PS-Simulink Converter3/1 -> [Tq_meas]
  connections:
  Torque Sensor/RConn1 -- C/RConn1
  Torque Sensor/RConn2 -- PS-Simulink Converter3/LConn1
  Torque Sensor/LConn1 -- R/RConn1

== system PMSMdetailTestbench/Test Environment ==
  In1 : Inport
  Break : Constant  Value=0
  Break1 : Constant
  Bus : Subsystem
  Road Inclination : Constant
  Switch : Switch  Criteria=u2 > Threshold  Threshold=-0.4557  SaturateOnIntegerOverflow=off  InputSameDT=off
  Wind Speed : Constant  Value=0
  b : Outport
  wires:
  Wind Speed/1 -> Bus/2(Wi)
  Bus/1(b) -> b/1
  Road Inclination/1 -> Bus/1(In)
  In1/1 -> Switch/2
  Switch/1 -> Bus/3(Br)
  Break/1 -> Switch/1
  Break1/1 -> Switch/3

== system PMSMdetailTestbench/Vehicle Dynamics ==
  Test data : Inport
  Brake Torque : Subsystem
  Bus Selector : BusSelector  OutputSignals=Incline,Wind speed,Brake pedal
  Drag and Gravity : Subsystem
  Force Source : fl_lib/Mechanical/Mechanical Sources/Ideal Force Source
  MTRef : fl_lib/Mechanical/Translational Elements/Mechanical Translational Reference
  PS Subtract1 : fl_ps_legacy_lib/Legacy Physical Signals/Functions/PS Subtract
  Sensing Speed : Subsystem
      mask Display: disp('v')
  Vehicle Mass : fl_lib/Mechanical/Translational Elements/Mass  mass=electricDrive.VehicleParams.vehicle_mass kg  num_ports=foundation.enum.numPorts2.one  v_specify=off  v_priority=High  v=0 m/s  v_nominal_specify=off  v_nominal_unit=m/s  v_nominal_value=1  f_specify=off  f_priority=High  f=0 N  f_nominal_specify=off  f_nominal_unit=N  f_nominal_value=1
  Wheel and Axle : fl_lib/Mechanical/Mechanisms/Wheel and Axle  R=electricDrive.VehicleParams.wheel_radius m  or=1  t_specify=off  t_priority=High  t=0 N*m  t_nominal_specify=off  t_nominal_unit=N*m  t_nominal_value=1  f_specify=off  f_priority=High  f=0 N  f_nominal_specify=off  f_nominal_unit=N  f_nominal_value=1
  R : PMIOPort  Side=Left
  wires:
  Test data/1 -> Bus Selector/1
  Bus Selector/3 -> Brake Torque/1(Pedal)  "<Brake pedal>"
  Bus Selector/1 -> Drag and Gravity/1(beta)  "<Incline>"
  Bus Selector/2 -> Drag and Gravity/2(vW)  "<Wind speed>"
  connections:
  Force Source/RConn2 -- MTRef/LConn1
  R/RConn1 -- Brake Torque/RConn1 -- Wheel and Axle/LConn1
  PS Subtract1/RConn1 -- Force Source/RConn1
  PS Subtract1/LConn1 -- Drag and Gravity/LConn3
  Drag and Gravity/LConn2 -- PS Subtract1/LConn2
  Wheel and Axle/RConn1 -- Sensing Speed/LConn1 -- Force Source/LConn1 -- Vehicle Mass/LConn1
  Sensing Speed/RConn1 -- Drag and Gravity/LConn1

== system PMSMdetailTestbench/ Motor Thermal/Air_HTC_calculation ==
  Rotor side  HTC : Subsystem
  Rotor_Taylor_Couette  HTC : Subsystem
  RPM : PMIOPort  Side=Left
  HTC1 : Outport
  HTC2 : Outport  Port=2
  wires:
  Rotor side  HTC/1(Output) -> HTC2/1
  Rotor_Taylor_Couette  HTC/1(Output) -> HTC1/1
  connections:
  Rotor side  HTC/LConn1 -- RPM/RConn1 -- Rotor_Taylor_Couette  HTC/LConn1

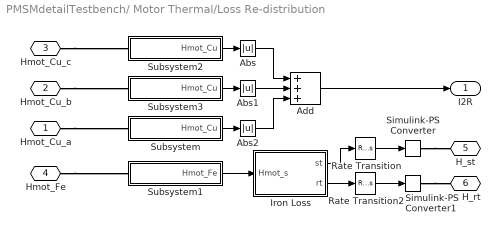
== system PMSMdetailTestbench/ Motor Thermal/Loss Re-distribution ==
  Abs : Abs  SaturateOnIntegerOverflow=off
  Abs1 : Abs  SaturateOnIntegerOverflow=off
  Abs2 : Abs  SaturateOnIntegerOverflow=off
  Add : Sum  Inputs=+++
  Iron Loss : Subsystem
  Rate Transition : RateTransition
  Rate Transition2 : RateTransition
  Simulink-PS Converter : nesl_utility/Simulink-PS Converter  PhysicalDomain=network_engine_domain  SubClassName=ps_input  LeftPortType=input  RightPortType=output  PseudoPeriodic=off  Frequencies=[]  NoiseDistribution=none  NoiseParameters=[]  Unit=W  AffineConversion=off  FilteringAndDerivatives=provide  SimscapeFilterOrder=1  InputFilterTimeConstant=0.001  UdotUserProvided=0
  Simulink-PS Converter1 : nesl_utility/Simulink-PS Converter  PhysicalDomain=network_engine_domain  SubClassName=ps_input  LeftPortType=input  RightPortType=output  PseudoPeriodic=off  Frequencies=[]  NoiseDistribution=none  NoiseParameters=[]  Unit=W  AffineConversion=off  FilteringAndDerivatives=provide  SimscapeFilterOrder=1  InputFilterTimeConstant=0.001  UdotUserProvided=0
  Subsystem : Subsystem
  Subsystem1 : Subsystem
  Subsystem2 : Subsystem
  Subsystem3 : Subsystem
  Hmot_Cu_a : PMIOPort  Side=Left
  Hmot_Cu_b : PMIOPort  Port=2  Side=Left
  Hmot_Cu_c : PMIOPort  Port=3  Side=Left
  Hmot_Fe : PMIOPort  Port=4  Side=Left
  H_st : PMIOPort  Port=5  Side=Right
  H_rt : PMIOPort  Port=6  Side=Right
  I2R : Outport
  wires:
  Subsystem1/1(Hmot_Fe) -> Iron Loss/1(Hmot_s)
  Iron Loss/1(st) -> Rate Transition/1
  Rate Transition/1 -> Simulink-PS Converter/1
  Iron Loss/2(rt) -> Rate Transition2/1
  Rate Transition2/1 -> Simulink-PS Converter1/1
  Add/1 -> I2R/1
  Subsystem2/1(Hmot_Cu) -> Abs/1
  Subsystem3/1(Hmot_Cu) -> Abs1/1
  Abs/1 -> Add/1
  Abs1/1 -> Add/2
  Subsystem/1(Hmot_Cu) -> Abs2/1
  Abs2/1 -> Add/3
  connections:
  Simulink-PS Converter/RConn1 -- H_st/RConn1
  Simulink-PS Converter1/RConn1 -- H_rt/RConn1
  Hmot_Cu_a/RConn1 -- Subsystem/LConn1
  Hmot_Fe/RConn1 -- Subsystem1/LConn1
  Hmot_Cu_c/RConn1 -- Subsystem2/LConn1
  Hmot_Cu_b/RConn1 -- Subsystem3/LConn1

== system PMSMdetailTestbench/ Motor Thermal/Speed Measurement ==
  Ideal Rotational Motion Sensor : fl_lib/Mechanical/Mechanical Sensors/Ideal Rotational Motion Sensor  reference=foundation.enum.MeasurementReference.difference  acceleration_port=false  velocity_port=true  position_port=true  wrap_angle=false  offset=0 rad
  MRRef1 : fl_lib/Mechanical/Rotational Elements/Mechanical Rotational Reference
  spd : PMIOPort  Side=Right
  mot : PMIOPort  Port=2  Side=Left
  connections:
  MRRef1/LConn1 -- Ideal Rotational Motion Sensor/RConn1
  mot/RConn1 -- Ideal Rotational Motion Sensor/LConn1
  spd/RConn1 -- Ideal Rotational Motion Sensor/RConn2

== system PMSMdetailTestbench/ Motor Thermal/Temperature ==
  I2R_Loss : Inport
  HTC1 : Inport  Port=2
  In1 : Inport  Port=3
  Rotor Thermal Block : Subsystem
      settings: PortSchema="{\"entries\":[{\"content\":{\"sides\":[{\"content\":{\"connectorIds\":[\"Out1\"]},\"type\":\"ConnectorPlacement.EquallySpacedRectSide\",\"uuid\":\"a0a486ff-95e2-43b7-8e3c-0cd0a05f759b\"},{\"content\":{\"connectorIds\":[\"RConn1\",\"In1\",\"In2\"],\"side\":\"RIGHT\"},\"type\":\"ConnectorPlacement.EquallySpacedRectSide\",\"uuid\":\"7508b6f9-91f5-4797-b9a6-d16ad4f8253e\"},{\"content\":{\"side\":\"TOP\"},\"type\":\"ConnectorPlacement.EquallySpacedRectSide\",\"uuid\":\"355558a4-f3bc-4897-a0c1-c168a45c32e0\"}]},\"type\":\"ConnectorPlacement.EquallySpacedConnector\",\"uuid\":\"a4aa0448-6fcb-4f55-be65-0b704c3933ab\"}],\"packageUris\":[\"http://schema.mathworks.com/mf0/Connector/R2020b\"],\"version\":\"1.0\"}"
  Stator Thermal Block : Subsystem
      settings: PortSchema="{\"entries\":[{\"content\":{\"sides\":[{\"content\":{\"connectorIds\":[\"LConn1\",\"Out1\"]},\"type\":\"ConnectorPlacement.EquallySpacedRectSide\",\"uuid\":\"dff33fed-3dc7-4aad-9227-94bf19dd06e3\"},{\"content\":{\"connectorIds\":[\"RConn1\",\"In1\"],\"side\":\"RIGHT\"},\"type\":\"ConnectorPlacement.EquallySpacedRectSide\",\"uuid\":\"142a0954-afc6-44e3-a8b1-fc5bc2b6a2e2\"},{\"content\":{\"side\":\"TOP\"},\"type\":\"ConnectorPlacement.EquallySpacedRectSide\",\"uuid\":\"7df235b3-e134-46ce-9adc-210f2635e5d6\"},{\"content\":{\"side\":\"BOTTOM\"},\"type\":\"ConnectorPlacement.EquallySpacedRectSide\",\"uuid\":\"bd40a8b4-b584-4f2f-8f49-bb9db9bb01e0\"}]},\"type\":\"ConnectorPlacement.EquallySpacedConnector\",\"uuid\":\"c512503b-3e59-4cb6-954f-d689dbce3646\"}],\"packageUris\":[\"http://schema.mathworks.com/mf0/Connector/R2020b\"],\"version\":\"1.0\"}"
  H_rt : PMIOPort  Side=Left
  H_st : PMIOPort  Port=2  Side=Left
  Hcoolant : PMIOPort  Port=3  Side=Right
  Twinding : Outport
  Tmagnet : Outport  Port=2
  wires:
  I2R_Loss/1 -> Stator Thermal Block/1(I2R_Loss)
  Stator Thermal Block/1(Output) -> Twinding/1
  Rotor Thermal Block/1(Output) -> Tmagnet/1
  In1/1 -> Rotor Thermal Block/1(In1)
  HTC1/1 -> Rotor Thermal Block/2(In2)
  connections:
  Hcoolant/RConn1 -- Stator Thermal Block/LConn1
  H_rt/RConn1 -- Rotor Thermal Block/RConn1
  H_st/RConn1 -- Stator Thermal Block/RConn1

== system PMSMdetailTestbench/Cooling System/Heat Exch. Characteristic ==
  Characteristic : Subsystem
  Heat Flow Source : fl_lib/Thermal/Thermal Sources/Controlled Heat Flow Rate Source
  Mass Flow Rate & Thermal Flux Sensor (TL) : fl_lib/Thermal Liquid/Sensors/Mass & Energy Flow Rate Sensor (TL)
      settings: InternalSimscapePortConfiguration="{\"Bottom\":[],\"Left\":[{\"id\":\"A\",\"label\":\"A\",\"type\":\"foundation.thermal_liquid.thermal_liquid\"}],\"Right\":[{\"id\":\"B\",\"label\":\"B\",\"type\":\"foundation.thermal_liquid.thermal_liquid\"},{\"id\":\"M\",\"label\":\"M\",\"type\":\"output\"},{\"id\":\"PHI\",\"label\":\"Phi\",\"type\":\"output\"}],\"Top\":[]}"
  Temperature Sensor : fl_lib/Thermal/Thermal Sensors/Temperature Sensor
  ThRef : fl_lib/Thermal/Thermal Elements/Thermal Reference
  Henv : PMIOPort  Side=Right
  Hp : PMIOPort  Port=2  Side=Left
  B : PMIOPort  Port=3  Side=Right
  Phi : PMIOPort  Port=4  Side=Right
  A : PMIOPort  Port=5  Side=Left
  T in : PMIOPort  Port=6  Side=Left
  connections:
  A/RConn1 -- Mass Flow Rate & Thermal Flux Sensor (TL)/LConn1
  Temperature Sensor/LConn1 -- Henv/RConn1 -- Heat Flow Source/RConn2
  ThRef/LConn1 -- Temperature Sensor/RConn1
  Heat Flow Source/LConn1 -- Hp/RConn1
  Mass Flow Rate & Thermal Flux Sensor (TL)/RConn1 -- B/RConn1
  Mass Flow Rate & Thermal Flux Sensor (TL)/RConn3 -- Phi/RConn1
  Mass Flow Rate & Thermal Flux Sensor (TL)/RConn2 -- Characteristic/RConn1
  T in/RConn1 -- Characteristic/RConn2
  Temperature Sensor/RConn2 -- Characteristic/RConn3
  Characteristic/LConn1 -- Heat Flow Source/RConn1
